simulink model "ConSys_A1"  (Simulink 8.3)
settings: Solver=ode3  StartTime=0.0  StopTime=Time(end)  FixedStep=Ts  RelTol=1e-3
values from neighbouring files (symbols this model uses):
  d = r*h    (= 1.6)    [StartUp_A1.m]
  d0 = d*h    (= 0.0032)    [StartUp_A1.m]
  h = 0.002    [StartUp_A1.m]
  Ka = diag([ 3  20  20  150  355  520])    [StartUp_A1.m]
  Kd = diag([ 3   5  25  100   15 1050])    [StartUp_A1.m]
  Ki = diag([35 555 810 7410 1850 5815])    [StartUp_A1.m]
  Kp = diag([55 180 350 1960  680 4450])    [StartUp_A1.m]
  r = 800    [StartUp_A1.m]
  TD = ss(Atd,Btd,Ctd,Dtd,Ts)    [StartUp_A1.m]
  Ts = 1/200    (= 0.005)    [StartUp_A1.m]
undefined symbols (not defined in the file or in its folder): DiscIntNeverNeededParam
undefined symbols (not defined in the file): ADAMS_cwd, ADAMS_exec, ADAMS_host, ADAMS_init, ADAMS_inputs, ADAMS_outputs, ADAMS_prefix, ADAMS_static, ADAMS_sysdir
libraries: cstblocks x6
(part 6 of 9)

== matlab function A2/MATLAB Function 3 ==
  data: q input double; V3 output double; dq input double
function V3 = V3(q,dq)
%#codegen
Th1=q(1,1); Th2=q(2,1); Th3=q(3,1); Th4=q(4,1); Th5=q(5,1); Th6=q(6,1);
dTh1=dq(1); dTh2=dq(2); dTh3=dq(3); dTh4=dq(4); dTh5=dq(5); dTh6=dq(6);
%---------------------------
V311=(1.3719*sin(2.0*Th2 + 2.0*Th3) - 0.006265*cos(2.0*Th2 + 2.0*Th3) + (0.01602*cos(Th2 + Th3) + 2.4568*sin(Th2 + Th3))*(0.13649*cos(Th2 + Th3) - 0.00089*sin(Th2 + Th3) + 0.36*sin(Th2) - 0.07) - 0.5*(cos(Th6)*(sin(Th2 + Th3)*sin(Th5) - 1.0*cos(Th2 + Th3)*cos(Th4)*cos(Th5)) + cos(Th2 + Th3)*sin(Th4)*sin(Th6))*(0.001043*cos(Th6)*(cos(Th2 + Th3)*sin(Th5) + sin(Th2 + Th3)*cos(Th4)*cos(Th5)) - 4.0e-6*cos(Th2 + Th3)*cos(Th5) + 4.0e-6*sin(Th2 + Th3)*cos(Th4)*sin(Th5) - 0.001043*sin(Th2 + Th3)*sin(Th4)*sin(Th6)) - 1.0*(0.126*sin(Th2 + Th3) + 0.00062*cos(Th2 + Th3)*sin(Th4) - 0.00152*sin(Th2 + Th3)*cos(Th5) - 0.00002*sin(Th2 + Th3)*sin(Th5) + 0.254*cos(Th2)*sin(Th3) + 0.254*cos(Th3)*sin(Th2) + 0.00002*cos(Th2 + Th3)*cos(Th4)*cos(Th5) - 0.00152*cos(Th2 + Th3)*cos(Th4)*sin(Th5))*(0.36*sin(Th2) - 0.126*cos(Th2 + Th3) + 0.00152*cos(Th2 + Th3)*cos(Th5) + 0.00002*cos(Th2 + Th3)*sin(Th5) + 0.00062*sin(Th2 + Th3)*sin(Th4) - 0.254*cos(Th2)*cos(Th3) + 0.254*sin(Th2)*sin(Th3) + 0.00002*sin(Th2 + Th3)*cos(Th4)*cos(Th5) - 0.00152*sin(Th2 + Th3)*cos(Th4)*sin(Th5) - 0.07) + (0.063*sin(Th2 + Th3) + 0.02603*sin(Th2 + Th3)*cos(Th5) + 0.127*cos(Th2)*sin(Th3) + 0.127*cos(Th3)*sin(Th2) + 0.02603*cos(Th2 + Th3)*cos(Th4)*sin(Th5) + 0.000115*cos(Th2 + Th3)*sin(Th4)*sin(Th6) + 0.000115*sin(Th2 + Th3)*cos(Th6)*sin(Th5) - 0.000115*cos(Th2 + Th3)*cos(Th4)*cos(Th5)*cos(Th6))*(0.126*cos(Th2 + Th3) - 0.36*sin(Th2) + 0.05206*cos(Th2 + Th3)*cos(Th5) + 0.254*cos(Th2)*cos(Th3) - 0.254*sin(Th2)*sin(Th3) + 0.00023*cos(Th2 + Th3)*cos(Th6)*sin(Th5) - 0.05206*sin(Th2 + Th3)*cos(Th4)*sin(Th5) - 0.00023*sin(Th2 + Th3)*sin(Th4)*sin(Th6) + 0.00023*sin(Th2 + Th3)*cos(Th4)*cos(Th5)*cos(Th6) + 0.07) - 0.004943*cos(Th2 + Th3)*sin(Th2 + Th3) - 0.5*(sin(Th6)*(cos(Th2 + Th3)*sin(Th5) + sin(Th2 + Th3)*cos(Th4)*cos(Th5)) + sin(Th2 + Th3)*cos(Th6)*sin(Th4))*(0.00104*sin(Th6)*(sin(Th2 + Th3)*sin(Th5) - 1.0*cos(Th2 + Th3)*cos(Th4)*cos(Th5)) - 0.00104*cos(Th2 + Th3)*cos(Th6)*sin(Th4)) - 0.5*(sin(Th6)*(sin(Th2 + Th3)*sin(Th5) - 1.0*cos(Th2 + Th3)*cos(Th4)*cos(Th5)) - 1.0*cos(Th2 + Th3)*cos(Th6)*sin(Th4))*(0.00104*sin(Th6)*(cos(Th2 + Th3)*sin(Th5) + sin(Th2 + Th3)*cos(Th4)*cos(Th5)) + 0.00104*sin(Th2 + Th3)*cos(Th6)*sin(Th4)) + 0.5*(sin(Th2 + Th3)*cos(Th5) + cos(Th2 + Th3)*cos(Th4)*sin(Th5))*(4.0e-6*cos(Th6)*(cos(Th2 + Th3)*sin(Th5) + sin(Th2 + Th3)*cos(Th4)*cos(Th5)) - 0.000116*cos(Th2 + Th3)*cos(Th5) + 0.000116*sin(Th2 + Th3)*cos(Th4)*sin(Th5) - 4.0e-6*sin(Th2 + Th3)*sin(Th4)*sin(Th6)) + 0.5*(cos(Th2 + Th3)*cos(Th5) - 1.0*sin(Th2 + Th3)*cos(Th4)*sin(Th5))*(4.0e-6*cos(Th6)*(sin(Th2 + Th3)*sin(Th5) - 1.0*cos(Th2 + Th3)*cos(Th4)*cos(Th5)) - 0.000116*sin(Th2 + Th3)*cos(Th5) - 0.000116*cos(Th2 + Th3)*cos(Th4)*sin(Th5) + 4.0e-6*cos(Th2 + Th3)*sin(Th4)*sin(Th6)) + (0.55399*sin(Th2 + Th3) + 1.651*cos(Th2)*sin(Th3) + 1.651*cos(Th3)*sin(Th2))*(0.08523*cos(Th2 + Th3) - 0.36*sin(Th2) + 0.254*cos(Th2)*cos(Th3) - 0.254*sin(Th2)*sin(Th3) + 0.07) - 0.5*(cos(Th6)*(cos(Th2 + Th3)*sin(Th5) + sin(Th2 + Th3)*cos(Th4)*cos(Th5)) - 1.0*sin(Th2 + Th3)*sin(Th4)*sin(Th6))*(0.001043*cos(Th6)*(sin(Th2 + Th3)*sin(Th5) - 1.0*cos(Th2 + Th3)*cos(Th4)*cos(Th5)) - 4.0e-6*sin(Th2 + Th3)*cos(Th5) - 4.0e-6*cos(Th2 + Th3)*cos(Th4)*sin(Th5) + 0.001043*cos(Th2 + Th3)*sin(Th4)*sin(Th6)) + 0.011125*cos(Th2 + Th3)*sin(Th2 + Th3)*cos(Th4)^2 - 0.000489*cos(Th2 + Th3)*sin(Th2 + Th3)*cos(Th5)^2 + 0.02091*cos(Th2 + Th3)*sin(Th2 + Th3)*sin(Th4)^2 - 0.004898*cos(Th2 + Th3)*sin(Th2 + Th3)*sin(Th5)^2 + 0.00004*cos(Th2 + Th3)^2*cos(Th5)*sin(Th4) - 0.00004*sin(Th2 + Th3)^2*cos(Th5)*sin(Th4) + 0.004409*cos(Th2 + Th3)^2*cos(Th4)*cos(Th5)*sin(Th5) - 0.004409*sin(Th2 + Th3)^2*cos(Th4)*cos(Th5)*sin(Th5) + 0.004898*cos(Th2 + Th3)*sin(Th2 + Th3)*cos(Th4)^2*cos(Th5)^2 + 0.000489*cos(Th2 + Th3)*sin(Th2 + Th3)*cos(Th4)^2*sin(Th5)^2 - 0.00008*cos(Th2 + Th3)*sin(Th2 + Th3)*cos(Th4)*sin(Th4)*sin(Th5))*dTh1*dTh1;
O312=0.019809*cos(Th2 + Th3) - 0.000076053*sin(Th2 + Th3) - 0.5*(0.00062*cos(Th4) - 0.00002*cos(Th5)*sin(Th4) + 0.00152*sin(Th4)*sin(Th5))*(0.00152*cos(Th2 + Th3)*cos(Th5) - 0.126*cos(Th2 + Th3) + 0.00002*cos(Th2 + Th3)*sin(Th5) + 0.00062*sin(Th2 + Th3)*sin(Th4) - 0.254*cos(Th2)*cos(Th3) + 0.254*sin(Th2)*sin(Th3) + 0.00002*sin(Th2 + Th3)*cos(Th4)*cos(Th5) - 0.00152*sin(Th2 + Th3)*cos(Th4)*sin(Th5)) + 0.00002*sin(Th2 + Th3)*sin(Th5) + 0.5*(0.000115*cos(Th4)*sin(Th6) - 0.02603*sin(Th4)*sin(Th5) + 0.000115*cos(Th5)*cos(Th6)*sin(Th4))*(0.126*cos(Th2 + Th3) + 0.05206*cos(Th2 + Th3)*cos(Th5) + 0.254*cos(Th2)*cos(Th3) - 0.254*sin(Th2)*sin(Th3) + 0.00023*cos(Th2 + Th3)*cos(Th6)*sin(Th5) - 0.05206*sin(Th2 + Th3)*cos(Th4)*sin(Th5) - 0.00023*sin(Th2 + Th3)*sin(Th4)*sin(Th6) + 0.00023*sin(Th2 + Th3)*cos(Th4)*cos(Th5)*cos(Th6)) + 0.00002*cos(Th2 + Th3)*cos(Th4)*cos(Th5) - 2.0e-6*cos(Th2 + Th3)*cos(Th6)*sin(Th4) + 0.0051115*sin(Th2 + Th3)*cos(Th4)*sin(Th4) + 2.0e-6*sin(Th2 + Th3)*sin(Th5)*sin(Th6) - 0.00004*sin(Th2 + Th3)*cos(Th4)^2*sin(Th5) + 2.0e-6*cos(Th2 + Th3)*cos(Th4)*cos(Th5)*sin(Th6) - 0.0026665*cos(Th2 + Th3)*cos(Th5)*sin(Th4)*sin(Th5) + 1.5e-6*sin(Th2 + Th3)*cos(Th5)*cos(Th6)*sin(Th6) + 4.0e-6*cos(Th2 + Th3)*cos(Th5)^2*cos(Th6)*sin(Th4) - 0.0026665*sin(Th2 + Th3)*cos(Th4)*cos(Th5)^2*sin(Th4) - 1.5e-6*sin(Th2 + Th3)*cos(Th4)*cos(Th6)^2*sin(Th4) - 4.0e-6*sin(Th2 + Th3)*cos(Th4)^2*sin(Th5)*sin(Th6) - 1.5e-6*cos(Th2 + Th3)*cos(Th5)*cos(Th6)^2*sin(Th4)*sin(Th5) - 3.0e-6*sin(Th2 + Th3)*cos(Th4)^2*cos(Th5)*cos(Th6)*sin(Th6) - 1.5e-6*sin(Th2 + Th3)*cos(Th4)*cos(Th5)^2*cos(Th6)^2*sin(Th4) - 1.5e-6*cos(Th2 + Th3)*cos(Th4)*cos(Th6)*sin(Th5)*sin(Th6) - 4.0e-6*sin(Th2 + Th3)*cos(Th4)*cos(Th5)*cos(Th6)*sin(Th4)*sin(Th5);
V312=O312*dTh1*dTh2;
V313=O312*dTh1*dTh3;
V314=(0.0054606*cos(Th2)*cos(Th3) - 0.0054606*sin(Th2)*sin(Th3) + 0.02316*cos(Th4)^2*sin(Th2)*sin(Th3) + 0.0033452*cos(Th5)^2*sin(Th2)*sin(Th3) + 4.4603e-6*cos(Th6)^2*sin(Th2)*sin(Th3) - 4.56e-8*cos(Th2)*cos(Th4)*sin(Th3) - 4.56e-8*cos(Th3)*cos(Th4)*sin(Th2) - 0.0003534*cos(Th2)*sin(Th3)*sin(Th4) - 0.0003534*cos(Th3)*sin(Th2)*sin(Th4) - 0.02316*cos(Th2)*cos(Th3)*cos(Th4)^2 - 0.0033452*cos(Th2)*cos(Th3)*cos(Th5)^2 - 4.4603e-6*cos(Th2)*cos(Th3)*cos(Th6)^2 - 0.013381*cos(Th4)^2*cos(Th5)^2*sin(Th2)*sin(Th3) - 5.9471e-6*cos(Th4)^2*cos(Th6)^2*sin(Th2)*sin(Th3) + 1.4868e-6*cos(Th5)^2*cos(Th6)^2*sin(Th2)*sin(Th3) - 0.0000114*cos(Th2)*cos(Th4)*cos(Th5)*sin(Th3) - 0.0000114*cos(Th3)*cos(Th4)*cos(Th5)*sin(Th2) - 3.04e-8*cos(Th2)*cos(Th3)*cos(Th5)*sin(Th5) - 0.00001498*cos(Th2)*cos(Th4)*cos(Th6)*sin(Th3) - 0.00001498*cos(Th3)*cos(Th4)*cos(Th6)*sin(Th2) - 0.013971*cos(Th2)*cos(Th4)*sin(Th3)*sin(Th5) - 0.000058586*cos(Th2)*cos(Th5)*sin(Th3)*sin(Th4) - 0.013971*cos(Th3)*cos(Th4)*sin(Th2)*sin(Th5) - 0.000058586*cos(Th3)*cos(Th5)*sin(Th2)*sin(Th4) + 1.86e-8*cos(Th2)*sin(Th3)*sin(Th4)*sin(Th5) + 1.86e-8*cos(Th3)*sin(Th2)*sin(Th4)*sin(Th5) - 0.00006555*cos(Th2)*sin(Th3)*sin(Th4)*sin(Th6) - 0.00006555*cos(Th3)*sin(Th2)*sin(Th4)*sin(Th6) + 3.04e-8*cos(Th5)*sin(Th2)*sin(Th3)*sin(Th5) + 9.12e-8*cos(Th2)*cos(Th4)*cos(Th5)^2*sin(Th3) + 9.12e-8*cos(Th3)*cos(Th4)*cos(Th5)^2*sin(Th2) + 0.013381*cos(Th2)*cos(Th3)*cos(Th4)^2*cos(Th5)^2 + 5.9471e-6*cos(Th2)*cos(Th3)*cos(Th4)^2*cos(Th6)^2 - 1.4868e-6*cos(Th2)*cos(Th3)*cos(Th5)^2*cos(Th6)^2 - 4.96e-8*cos(Th2)*cos(Th3)*cos(Th4)*cos(Th5)*sin(Th4) + 0.00006555*cos(Th2)*cos(Th4)*cos(Th5)*cos(Th6)*sin(Th3) + 0.00006555*cos(Th3)*cos(Th4)*cos(Th5)*cos(Th6)*sin(Th2) - 9.9869e-6*cos(Th2)*cos(Th3)*cos(Th5)*cos(Th6)*sin(Th5) + 5.9471e-6*cos(Th2)*cos(Th3)*cos(Th4)^2*cos(Th5)^2*cos(Th6)^2 - 0.00015623*cos(Th2)*cos(Th3)*cos(Th4)*sin(Th4)*sin(Th5) - 0.010036*cos(Th2)*cos(Th4)*cos(Th5)*sin(Th3)*sin(Th5) - 0.010036*cos(Th3)*cos(Th4)*cos(Th5)*sin(Th2)*sin(Th5) + 4.96e-8*cos(Th4)*cos(Th5)*sin(Th2)*sin(Th3)*sin(Th4) - 0.00001498*cos(Th2)*cos(Th5)*sin(Th3)*sin(Th4)*sin(Th6) - 0.00001498*cos(Th3)*cos(Th5)*sin(Th2)*sin(Th4)*sin(Th6) + 9.9869e-6*cos(Th5)*cos(Th6)*sin(Th2)*sin(Th3)*sin(Th5) - 5.9471e-6*cos(Th4)^2*cos(Th5)^2*cos(Th6)^2*sin(Th2)*sin(Th3) + 0.00015623*cos(Th4)*sin(Th2)*sin(Th3)*sin(Th4)*sin(Th5) + 1.216e-7*cos(Th2)*cos(Th3)*cos(Th4)^2*cos(Th5)*sin(Th5) + 0.000029961*cos(Th2)*cos(Th4)*cos(Th5)^2*cos(Th6)*sin(Th3) + 0.000029961*cos(Th3)*cos(Th4)*cos(Th5)^2*cos(Th6)*sin(Th2) - 1.216e-7*cos(Th4)^2*cos(Th5)*sin(Th2)*sin(Th3)*sin(Th5) + 0.000039948*cos(Th2)*cos(Th3)*cos(Th4)^2*cos(Th5)*cos(Th6)*sin(Th5) - 4.4603e-6*cos(Th2)*cos(Th4)*cos(Th5)*cos(Th6)^2*sin(Th3)*sin(Th5) - 4.4603e-6*cos(Th3)*cos(Th4)*cos(Th5)*cos(Th6)^2*sin(Th2)*sin(Th5) - 0.000039948*cos(Th4)^2*cos(Th5)*cos(Th6)*sin(Th2)*sin(Th3)*sin(Th5) - 0.000039948*cos(Th2)*cos(Th3)*cos(Th4)*sin(Th4)*sin(Th5)*sin(Th6) + 4.4603e-6*cos(Th2)*cos(Th6)*sin(Th3)*sin(Th4)*sin(Th5)*sin(Th6) + 4.4603e-6*cos(Th3)*cos(Th6)*sin(Th2)*sin(Th4)*sin(Th5)*sin(Th6) + 0.000039948*cos(Th4)*sin(Th2)*sin(Th3)*sin(Th4)*sin(Th5)*sin(Th6) - 0.000011894*cos(Th2)*cos(Th3)*cos(Th4)*cos(Th5)*cos(Th6)*sin(Th4)*sin(Th6) + 0.000011894*cos(Th4)*cos(Th5)*cos(Th6)*sin(Th2)*sin(Th3)*sin(Th4)*sin(Th6))*dTh1*dTh4;
V315=(1.86e-8*cos(Th2)*cos(Th3)*sin(Th5) - 0.000058586*cos(Th2)*cos(Th3)*cos(Th5) + 0.0028942*cos(Th2)*sin(Th3)*sin(Th4) + 0.0028942*cos(Th3)*sin(Th2)*sin(Th4) + 0.000058586*cos(Th5)*sin(Th2)*sin(Th3) - 1.86e-8*sin(Th2)*sin(Th3)*sin(Th5) - 6.08e-8*cos(Th2)*cos(Th3)*cos(Th4)*sin(Th4) - 6.2e-9*cos(Th2)*cos(Th4)*cos(Th5)*sin(Th3) - 6.2e-9*cos(Th3)*cos(Th4)*cos(Th5)*sin(Th2) - 0.00001498*cos(Th2)*cos(Th3)*cos(Th5)*sin(Th6) - 0.000019529*cos(Th2)*cos(Th4)*sin(Th3)*sin(Th5) - 0.013971*cos(Th2)*cos(Th5)*sin(Th3)*sin(Th4) - 0.000019529*cos(Th3)*cos(Th4)*sin(Th2)*sin(Th5) - 0.013971*cos(Th3)*cos(Th5)*sin(Th2)*sin(Th4) + 6.08e-8*cos(Th4)*sin(Th2)*sin(Th3)*sin(Th4) + 0.0000114*cos(Th2)*sin(Th3)*sin(Th4)*sin(Th5) + 0.0000114*cos(Th3)*sin(Th2)*sin(Th4)*sin(Th5) + 0.00001498*cos(Th5)*sin(Th2)*sin(Th3)*sin(Th6) + 0.000078115*cos(Th2)*cos(Th3)*cos(Th4)^2*cos(Th5) - 2.48e-8*cos(Th2)*cos(Th3)*cos(Th4)^2*sin(Th5) - 0.013381*cos(Th2)*cos(Th5)^2*sin(Th3)*sin(Th4) - 0.013381*cos(Th3)*cos(Th5)^2*sin(Th2)*sin(Th4) - 0.000078115*cos(Th4)^2*cos(Th5)*sin(Th2)*sin(Th3) + 4.4603e-6*cos(Th2)*cos(Th6)^2*sin(Th3)*sin(Th4) + 4.4603e-6*cos(Th3)*cos(Th6)^2*sin(Th2)*sin(Th4) + 2.48e-8*cos(Th4)^2*sin(Th2)*sin(Th3)*sin(Th5) - 0.000019974*cos(Th2)*cos(Th3)*cos(Th4)*cos(Th6)*sin(Th4) + 4.4603e-6*cos(Th2)*cos(Th3)*cos(Th6)*sin(Th5)*sin(Th6) - 1.216e-7*cos(Th2)*cos(Th5)*sin(Th3)*sin(Th4)*sin(Th5) - 1.216e-7*cos(Th3)*cos(Th5)*sin(Th2)*sin(Th4)*sin(Th5) + 0.000019974*cos(Th4)*cos(Th6)*sin(Th2)*sin(Th3)*sin(Th4) - 4.9934e-6*cos(Th2)*cos(Th4)*sin(Th3)*sin(Th5)*sin(Th6) - 0.00006555*cos(Th2)*cos(Th6)*sin(Th3)*sin(Th4)*sin(Th5) - 4.9934e-6*cos(Th3)*cos(Th4)*sin(Th2)*sin(Th5)*sin(Th6) - 0.00006555*cos(Th3)*cos(Th6)*sin(Th2)*sin(Th4)*sin(Th5) - 4.4603e-6*cos(Th6)*sin(Th2)*sin(Th3)*sin(Th5)*sin(Th6) + 1.216e-7*cos(Th2)*cos(Th3)*cos(Th4)*cos(Th5)^2*sin(Th4) + 0.000019974*cos(Th2)*cos(Th3)*cos(Th4)^2*cos(Th5)*sin(Th6) - 1.216e-7*cos(Th4)*cos(Th5)^2*sin(Th2)*sin(Th3)*sin(Th4) - 0.000019974*cos(Th4)^2*cos(Th5)*sin(Th2)*sin(Th3)*sin(Th6) - 5.9471e-6*cos(Th2)*cos(Th5)^2*cos(Th6)^2*sin(Th3)*sin(Th4) - 5.9471e-6*cos(Th3)*cos(Th5)^2*cos(Th6)^2*sin(Th2)*sin(Th4) + 0.000039948*cos(Th2)*cos(Th3)*cos(Th4)*cos(Th5)^2*cos(Th6)*sin(Th4) - 5.9471e-6*cos(Th2)*cos(Th3)*cos(Th4)^2*cos(Th6)*sin(Th5)*sin(Th6) - 0.000039948*cos(Th4)*cos(Th5)^2*cos(Th6)*sin(Th2)*sin(Th3)*sin(Th4) + 5.9471e-6*cos(Th4)^2*cos(Th6)*sin(Th2)*sin(Th3)*sin(Th5)*sin(Th6) - 0.013381*cos(Th2)*cos(Th3)*cos(Th4)*cos(Th5)*sin(Th4)*sin(Th5) - 1.4868e-6*cos(Th2)*cos(Th4)*cos(Th5)*cos(Th6)*sin(Th3)*sin(Th6) - 1.4868e-6*cos(Th3)*cos(Th4)*cos(Th5)*cos(Th6)*sin(Th2)*sin(Th6) - 0.000039948*cos(Th2)*cos(Th5)*cos(Th6)*sin(Th3)*sin(Th4)*sin(Th5) - 0.000039948*cos(Th3)*cos(Th5)*cos(Th6)*sin(Th2)*sin(Th4)*sin(Th5) + 0.013381*cos(Th4)*cos(Th5)*sin(Th2)*sin(Th3)*sin(Th4)*sin(Th5) + 5.9471e-6*cos(Th4)*cos(Th5)*cos(Th6)^2*sin(Th2)*sin(Th3)*sin(Th4)*sin(Th5) - 5.9471e-6*cos(Th2)*cos(Th3)*cos(Th4)*cos(Th5)*cos(Th6)^2*sin(Th4)*sin(Th5))*dTh1*dTh5;
V316=(0.00005504*cos(Th5)*sin(Th2)*sin(Th3) - 0.00005504*cos(Th2)*cos(Th3)*cos(Th5) + 0.00006555*cos(Th2)*cos(Th4)*cos(Th6)*sin(Th3) + 0.00006555*cos(Th3)*cos(Th4)*cos(Th6)*sin(Th2) - 4.9934e-6*cos(Th2)*cos(Th3)*cos(Th6)*sin(Th5) + 0.000060987*cos(Th2)*cos(Th4)*sin(Th3)*sin(Th5) + 0.000060987*cos(Th3)*cos(Th4)*sin(Th2)*sin(Th5) + 4.9934e-6*cos(Th2)*sin(Th3)*sin(Th4)*sin(Th6) + 4.9934e-6*cos(Th3)*sin(Th2)*sin(Th4)*sin(Th6) + 4.9934e-6*cos(Th6)*sin(Th2)*sin(Th3)*sin(Th5) - 5.9471e-6*cos(Th2)*cos(Th3)*cos(Th4)^2*cos(Th5) - 5.9471e-6*cos(Th2)*cos(Th3)*cos(Th5)*cos(Th6)^2 + 5.9471e-6*cos(Th4)^2*cos(Th5)*sin(Th2)*sin(Th3) + 5.9471e-6*cos(Th5)*cos(Th6)^2*sin(Th2)*sin(Th3) + 0.00001498*cos(Th2)*cos(Th4)*cos(Th5)*cos(Th6)*sin(Th3) + 0.00001498*cos(Th3)*cos(Th4)*cos(Th5)*cos(Th6)*sin(Th2) - 0.00006555*cos(Th2)*cos(Th5)*sin(Th3)*sin(Th4)*sin(Th6) - 0.00006555*cos(Th3)*cos(Th5)*sin(Th2)*sin(Th4)*sin(Th6) + 0.000019974*cos(Th2)*cos(Th3)*cos(Th4)^2*cos(Th6)*sin(Th5) - 5.9471e-6*cos(Th2)*cos(Th4)*cos(Th6)^2*sin(Th3)*sin(Th5) - 5.9471e-6*cos(Th3)*cos(Th4)*cos(Th6)^2*sin(Th2)*sin(Th5) - 0.000019974*cos(Th2)*cos(Th5)^2*sin(Th3)*sin(Th4)*sin(Th6) - 0.000019974*cos(Th3)*cos(Th5)^2*sin(Th2)*sin(Th4)*sin(Th6) - 0.000019974*cos(Th4)^2*cos(Th6)*sin(Th2)*sin(Th3)*sin(Th5) + 0.000011894*cos(Th2)*cos(Th3)*cos(Th4)^2*cos(Th5)*cos(Th6)^2 - 0.000011894*cos(Th4)^2*cos(Th5)*cos(Th6)^2*sin(Th2)*sin(Th3) - 5.9471e-6*cos(Th2)*cos(Th3)*cos(Th4)*cos(Th6)*sin(Th4)*sin(Th6) + 5.9471e-6*cos(Th4)*cos(Th6)*sin(Th2)*sin(Th3)*sin(Th4)*sin(Th6) + 5.9471e-6*cos(Th4)*cos(Th5)^2*cos(Th6)*sin(Th2)*sin(Th3)*sin(Th4)*sin(Th6) - 0.000019974*cos(Th2)*cos(Th3)*cos(Th4)*cos(Th5)*sin(Th4)*sin(Th5)*sin(Th6) + 5.9471e-6*cos(Th2)*cos(Th5)*cos(Th6)*sin(Th3)*sin(Th4)*sin(Th5)*sin(Th6) + 5.9471e-6*cos(Th3)*cos(Th5)*cos(Th6)*sin(Th2)*sin(Th4)*sin(Th5)*sin(Th6) + 0.000019974*cos(Th4)*cos(Th5)*sin(Th2)*sin(Th3)*sin(Th4)*sin(Th5)*sin(Th6) - 5.9471e-6*cos(Th2)*cos(Th3)*cos(Th4)*cos(Th5)^2*cos(Th6)*sin(Th4)*sin(Th6))*dTh1*dTh6;
%---------------------------
V321=(0.000076053*sin(Th2 + Th3) - 0.019809*cos(Th2 + Th3) + 0.5*(0.00062*cos(Th4) - 0.00002*cos(Th5)*sin(Th4) + 0.00152*sin(Th4)*sin(Th5))*(0.00152*cos(Th2 + Th3)*cos(Th5) - 0.126*cos(Th2 + Th3) + 0.00002*cos(Th2 + Th3)*sin(Th5) + 0.00062*sin(Th2 + Th3)*sin(Th4) - 0.254*cos(Th2)*cos(Th3) + 0.254*sin(Th2)*sin(Th3) + 0.00002*sin(Th2 + Th3)*cos(Th4)*cos(Th5) - 0.00152*sin(Th2 + Th3)*cos(Th4)*sin(Th5)) - 0.00002*sin(Th2 + Th3)*sin(Th5) - 0.5*(0.000115*cos(Th4)*sin(Th6) - 0.02603*sin(Th4)*sin(Th5) + 0.000115*cos(Th5)*cos(Th6)*sin(Th4))*(0.126*cos(Th2 + Th3) + 0.05206*cos(Th2 + Th3)*cos(Th5) + 0.254*cos(Th2)*cos(Th3) - 0.254*sin(Th2)*sin(Th3) + 0.00023*cos(Th2 + Th3)*cos(Th6)*sin(Th5) - 0.05206*sin(Th2 + Th3)*cos(Th4)*sin(Th5) - 0.00023*sin(Th2 + Th3)*sin(Th4)*sin(Th6) + 0.00023*sin(Th2 + Th3)*cos(Th4)*cos(Th5)*cos(Th6)) - 0.00002*cos(Th2 + Th3)*cos(Th4)*cos(Th5) + 2.0e-6*cos(Th2 + Th3)*cos(Th6)*sin(Th4) - 0.0051115*sin(Th2 + Th3)*cos(Th4)*sin(Th4) - 2.0e-6*sin(Th2 + Th3)*sin(Th5)*sin(Th6) + 0.00004*sin(Th2 + Th3)*cos(Th4)^2*sin(Th5) - 2.0e-6*cos(Th2 + Th3)*cos(Th4)*cos(Th5)*sin(Th6) + 0.0026665*cos(Th2 + Th3)*cos(Th5)*sin(Th4)*sin(Th5) - 1.5e-6*sin(Th2 + Th3)*cos(Th5)*cos(Th6)*sin(Th6) - 4.0e-6*cos(Th2 + Th3)*cos(Th5)^2*cos(Th6)*sin(Th4) + 0.0026665*sin(Th2 + Th3)*cos(Th4)*cos(Th5)^2*sin(Th4) + 1.5e-6*sin(Th2 + Th3)*cos(Th4)*cos(Th6)^2*sin(Th4) + 4.0e-6*sin(Th2 + Th3)*cos(Th4)^2*sin(Th5)*sin(Th6) + 1.5e-6*cos(Th2 + Th3)*cos(Th5)*cos(Th6)^2*sin(Th4)*sin(Th5) + 3.0e-6*sin(Th2 + Th3)*cos(Th4)^2*cos(Th5)*cos(Th6)*sin(Th6) + 1.5e-6*sin(Th2 + Th3)*cos(Th4)*cos(Th5)^2*cos(Th6)^2*sin(Th4) + 1.5e-6*cos(Th2 + Th3)*cos(Th4)*cos(Th6)*sin(Th5)*sin(Th6) + 4.0e-6*sin(Th2 + Th3)*cos(Th4)*cos(Th5)*cos(Th6)*sin(Th4)*sin(Th5))*dTh2*dTh1;
V322=(7.2e-6*cos(Th3)*sin(Th5) - 0.0057672*sin(Th3) - 0.0088236*cos(Th3)*cos(Th5) - 0.11454*cos(Th3) + 0.0002232*sin(Th3)*sin(Th4) + 7.2e-6*cos(Th4)*cos(Th5)*sin(Th3) - 0.0000414*cos(Th3)*cos(Th6)*sin(Th5) + 0.0088236*cos(Th4)*sin(Th3)*sin(Th5) + 0.0000414*sin(Th3)*sin(Th4)*sin(Th6) - 0.0000414*cos(Th4)*cos(Th5)*cos(Th6)*sin(Th3))*dTh2*dTh2;
V323=(0.057271*cos(Th3) + 0.0028836*sin(Th3) + 0.0044118*cos(Th3)*cos(Th5) - 3.6e-6*cos(Th3)*sin(Th5) - 0.0001116*sin(Th3)*sin(Th4) - 3.6e-6*cos(Th4)*cos(Th5)*sin(Th3) + 0.0000207*cos(Th3)*cos(Th6)*sin(Th5) - 0.0044118*cos(Th4)*sin(Th3)*sin(Th5) - 0.0000207*sin(Th3)*sin(Th4)*sin(Th6) + 0.0000207*cos(Th4)*cos(Th5)*cos(Th6)*sin(Th3))*dTh2*dTh3;
V324=(4.96e-8*cos(Th4)^2*cos(Th5) - 2.48e-8*cos(Th5) - 0.000078115*sin(Th5) - 0.01158*sin(2.0*Th4) + 0.00015623*cos(Th4)^2*sin(Th5) + 0.0001116*cos(Th3)*cos(Th4) - 0.000019974*sin(Th5)*sin(Th6) + 0.000039948*cos(Th4)^2*sin(Th5)*sin(Th6) - 3.6e-6*cos(Th3)*cos(Th5)*sin(Th4) + 0.0000207*cos(Th3)*cos(Th4)*sin(Th6) - 5.9471e-6*cos(Th5)*cos(Th6)*sin(Th6) - 0.0044118*cos(Th3)*sin(Th4)*sin(Th5) + 0.013381*cos(Th4)*cos(Th5)^2*sin(Th4) + 5.9471e-6*cos(Th4)*cos(Th6)^2*sin(Th4) + 5.9471e-6*cos(Th4)*cos(Th5)^2*cos(Th6)^2*sin(Th4) + 0.0000207*cos(Th3)*cos(Th5)*cos(Th6)*sin(Th4) + 1.216e-7*cos(Th4)*cos(Th5)*sin(Th4)*sin(Th5) + 0.000011894*cos(Th4)^2*cos(Th5)*cos(Th6)*sin(Th6) + 0.000039948*cos(Th4)*cos(Th5)*cos(Th6)*sin(Th4)*sin(Th5))*dTh2*dTh4;
V325=(6.08e-8*cos(Th4)^2 - 0.0000152*cos(Th5) - 0.000019974*cos(Th6) - 0.018628*sin(Th5) - 0.0066904*sin(2.0*Th5) + 1.216e-7*cos(Th5)^2 + 0.000019974*cos(Th4)^2*cos(Th6) + 0.000039948*cos(Th5)^2*cos(Th6) - 1.216e-7*cos(Th4)^2*cos(Th5)^2 + 0.0000874*cos(Th5)*cos(Th6) - 3.6e-6*cos(Th5)*sin(Th3) - 0.0044118*sin(Th3)*sin(Th5) - 0.000039948*cos(Th4)^2*cos(Th5)^2*cos(Th6) + 0.0044118*cos(Th3)*cos(Th4)*cos(Th5) - 3.6e-6*cos(Th3)*cos(Th4)*sin(Th5) + 0.000078115*cos(Th4)*cos(Th5)*sin(Th4) + 0.0000207*cos(Th5)*cos(Th6)*sin(Th3) - 2.48e-8*cos(Th4)*sin(Th4)*sin(Th5) + 0.013381*cos(Th4)^2*cos(Th5)*sin(Th5) - 5.9471e-6*cos(Th5)*cos(Th6)^2*sin(Th5) + 5.9471e-6*cos(Th4)^2*cos(Th5)*cos(Th6)^2*sin(Th5) + 0.0000207*cos(Th3)*cos(Th4)*cos(Th6)*sin(Th5) + 0.000019974*cos(Th4)*cos(Th5)*sin(Th4)*sin(Th6) - 5.9471e-6*cos(Th4)*cos(Th6)*sin(Th4)*sin(Th5)*sin(Th6) - 6.08e-8)*dTh2*dTh5;
V326=(0.0000207*cos(Th3)*cos(Th6)*sin(Th4) - 0.0000874*sin(Th5)*sin(Th6) - 5.9471e-6*cos(Th4)*cos(Th5)*sin(Th4) - 0.000019974*cos(Th5)*sin(Th5)*sin(Th6) - 0.0000207*sin(Th3)*sin(Th5)*sin(Th6) + 5.9471e-6*cos(Th4)^2*cos(Th6)*sin(Th6) - 5.9471e-6*cos(Th5)^2*cos(Th6)*sin(Th6) + 5.9471e-6*cos(Th4)^2*cos(Th5)^2*cos(Th6)*sin(Th6) + 0.0000207*cos(Th3)*cos(Th4)*cos(Th5)*sin(Th6) + 0.000019974*cos(Th4)*cos(Th6)*sin(Th4)*sin(Th5) + 0.000011894*cos(Th4)*cos(Th5)*cos(Th6)^2*sin(Th4) + 0.000019974*cos(Th4)^2*cos(Th5)*sin(Th5)*sin(Th6))*dTh2*dTh6;
%---------------------------
V331=(0.000076053*sin(Th2 + Th3) - 0.019809*cos(Th2 + Th3) + 0.5*(0.00062*cos(Th4) - 0.00002*cos(Th5)*sin(Th4) + 0.00152*sin(Th4)*sin(Th5))*(0.00152*cos(Th2 + Th3)*cos(Th5) - 0.126*cos(Th2 + Th3) + 0.00002*cos(Th2 + Th3)*sin(Th5) + 0.00062*sin(Th2 + Th3)*sin(Th4) - 0.254*cos(Th2)*cos(Th3) + 0.254*sin(Th2)*sin(Th3) + 0.00002*sin(Th2 + Th3)*cos(Th4)*cos(Th5) - 0.00152*sin(Th2 + Th3)*cos(Th4)*sin(Th5)) - 0.00002*sin(Th2 + Th3)*sin(Th5) - 0.5*(0.000115*cos(Th4)*sin(Th6) - 0.02603*sin(Th4)*sin(Th5) + 0.000115*cos(Th5)*cos(Th6)*sin(Th4))*(0.126*cos(Th2 + Th3) + 0.05206*cos(Th2 + Th3)*cos(Th5) + 0.254*cos(Th2)*cos(Th3) - 0.254*sin(Th2)*sin(Th3) + 0.00023*cos(Th2 + Th3)*cos(Th6)*sin(Th5) - 0.05206*sin(Th2 + Th3)*cos(Th4)*sin(Th5) - 0.00023*sin(Th2 + Th3)*sin(Th4)*sin(Th6) + 0.00023*sin(Th2 + Th3)*cos(Th4)*cos(Th5)*cos(Th6)) - 0.00002*cos(Th2 + Th3)*cos(Th4)*cos(Th5) + 2.0e-6*cos(Th2 + Th3)*cos(Th6)*sin(Th4) - 0.0051115*sin(Th2 + Th3)*cos(Th4)*sin(Th4) - 2.0e-6*sin(Th2 + Th3)*sin(Th5)*sin(Th6) + 0.00004*sin(Th2 + Th3)*cos(Th4)^2*sin(Th5) - 2.0e-6*cos(Th2 + Th3)*cos(Th4)*cos(Th5)*sin(Th6) + 0.0026665*cos(Th2 + Th3)*cos(Th5)*sin(Th4)*sin(Th5) - 1.5e-6*sin(Th2 + Th3)*cos(Th5)*cos(Th6)*sin(Th6) - 4.0e-6*cos(Th2 + Th3)*cos(Th5)^2*cos(Th6)*sin(Th4) + 0.0026665*sin(Th2 + Th3)*cos(Th4)*cos(Th5)^2*sin(Th4) + 1.5e-6*sin(Th2 + Th3)*cos(Th4)*cos(Th6)^2*sin(Th4) + 4.0e-6*sin(Th2 + Th3)*cos(Th4)^2*sin(Th5)*sin(Th6) + 1.5e-6*cos(Th2 + Th3)*cos(Th5)*cos(Th6)^2*sin(Th4)*sin(Th5) + 3.0e-6*sin(Th2 + Th3)*cos(Th4)^2*cos(Th5)*cos(Th6)*sin(Th6) + 1.5e-6*sin(Th2 + Th3)*cos(Th4)*cos(Th5)^2*cos(Th6)^2*sin(Th4) + 1.5e-6*cos(Th2 + Th3)*cos(Th4)*cos(Th6)*sin(Th5)*sin(Th6) + 4.0e-6*sin(Th2 + Th3)*cos(Th4)*cos(Th5)*cos(Th6)*sin(Th4)*sin(Th5))*dTh3*dTh1;
V332=(3.6e-6*cos(Th3)*sin(Th5) - 0.0028836*sin(Th3) - 0.0044118*cos(Th3)*cos(Th5) - 0.057271*cos(Th3) + 0.0001116*sin(Th3)*sin(Th4) + 3.6e-6*cos(Th4)*cos(Th5)*sin(Th3) - 0.0000207*cos(Th3)*cos(Th6)*sin(Th5) + 0.0044118*cos(Th4)*sin(Th3)*sin(Th5) + 0.0000207*sin(Th3)*sin(Th4)*sin(Th6) - 0.0000207*cos(Th4)*cos(Th5)*cos(Th6)*sin(Th3))*dTh3*dTh2;
V333=(0)*dTh3*dTh3;
V334=(4.96e-8*cos(Th4)^2*cos(Th5) - 2.48e-8*cos(Th5) - 0.000078115*sin(Th5) - 0.01158*sin(2.0*Th4) + 0.00015623*cos(Th4)^2*sin(Th5) - 0.000019974*sin(Th5)*sin(Th6) + 0.000039948*cos(Th4)^2*sin(Th5)*sin(Th6) - 5.9471e-6*cos(Th5)*cos(Th6)*sin(Th6) + 0.013381*cos(Th4)*cos(Th5)^2*sin(Th4) + 5.9471e-6*cos(Th4)*cos(Th6)^2*sin(Th4) + 5.9471e-6*cos(Th4)*cos(Th5)^2*cos(Th6)^2*sin(Th4) + 1.216e-7*cos(Th4)*cos(Th5)*sin(Th4)*sin(Th5) + 0.000011894*cos(Th4)^2*cos(Th5)*cos(Th6)*sin(Th6) + 0.000039948*cos(Th4)*cos(Th5)*cos(Th6)*sin(Th4)*sin(Th5))*dTh3*dTh4;
V335=(6.08e-8*cos(Th4)^2 - 0.0000152*cos(Th5) - 0.000019974*cos(Th6) - 0.018628*sin(Th5) - 0.0066904*sin(2.0*Th5) + 1.216e-7*cos(Th5)^2 + 0.000019974*cos(Th4)^2*cos(Th6) + 0.000039948*cos(Th5)^2*cos(Th6) - 1.216e-7*cos(Th4)^2*cos(Th5)^2 + 0.0000874*cos(Th5)*cos(Th6) - 0.000039948*cos(Th4)^2*cos(Th5)^2*cos(Th6) + 0.000078115*cos(Th4)*cos(Th5)*sin(Th4) - 2.48e-8*cos(Th4)*sin(Th4)*sin(Th5) + 0.013381*cos(Th4)^2*cos(Th5)*sin(Th5) - 5.9471e-6*cos(Th5)*cos(Th6)^2*sin(Th5) + 5.9471e-6*cos(Th4)^2*cos(Th5)*cos(Th6)^2*sin(Th5) + 0.000019974*cos(Th4)*cos(Th5)*sin(Th4)*sin(Th6) - 5.9471e-6*cos(Th4)*cos(Th6)*sin(Th4)*sin(Th5)*sin(Th6) - 6.08e-8)*dTh3*dTh5;
V336=(5.9471e-6*cos(Th4)^2*cos(Th6)*sin(Th6) - 5.9471e-6*cos(Th4)*cos(Th5)*sin(Th4) - 0.000019974*cos(Th5)*sin(Th5)*sin(Th6) - 0.0000874*sin(Th5)*sin(Th6) - 5.9471e-6*cos(Th5)^2*cos(Th6)*sin(Th6) + 5.9471e-6*cos(Th4)^2*cos(Th5)^2*cos(Th6)*sin(Th6) + 0.000019974*cos(Th4)*cos(Th6)*sin(Th4)*sin(Th5) + 0.000011894*cos(Th4)*cos(Th5)*cos(Th6)^2*sin(Th4) + 0.000019974*cos(Th4)^2*cos(Th5)*sin(Th5)*sin(Th6))*dTh3*dTh6;
%---------------------------
V341=(0.0061194*sin(Th2)*sin(Th3) - 0.0061194*cos(Th2)*cos(Th3) - 0.0033452*cos(Th5)^2*sin(Th2)*sin(Th3) + 1.4868e-6*cos(Th6)^2*sin(Th2)*sin(Th3) - 1.52e-8*cos(Th2)*cos(Th4)*sin(Th3) - 1.52e-8*cos(Th3)*cos(Th4)*sin(Th2) - 0.0001178*cos(Th2)*sin(Th3)*sin(Th4) - 0.0001178*cos(Th3)*sin(Th2)*sin(Th4) + 0.0033452*cos(Th2)*cos(Th3)*cos(Th5)^2 - 1.4868e-6*cos(Th2)*cos(Th3)*cos(Th6)^2 - 1.4868e-6*cos(Th5)^2*cos(Th6)^2*sin(Th2)*sin(Th3) - 3.8e-6*cos(Th2)*cos(Th4)*cos(Th5)*sin(Th3) - 3.8e-6*cos(Th3)*cos(Th4)*cos(Th5)*sin(Th2) + 3.04e-8*cos(Th2)*cos(Th3)*cos(Th5)*sin(Th5) - 4.9934e-6*cos(Th2)*cos(Th4)*cos(Th6)*sin(Th3) - 4.9934e-6*cos(Th3)*cos(Th4)*cos(Th6)*sin(Th2) - 0.0046569*cos(Th2)*cos(Th4)*sin(Th3)*sin(Th5) - 0.000019529*cos(Th2)*cos(Th5)*sin(Th3)*sin(Th4) - 0.0046569*cos(Th3)*cos(Th4)*sin(Th2)*sin(Th5) - 0.000019529*cos(Th3)*cos(Th5)*sin(Th2)*sin(Th4) + 6.2e-9*cos(Th2)*sin(Th3)*sin(Th4)*sin(Th5) + 6.2e-9*cos(Th3)*sin(Th2)*sin(Th4)*sin(Th5) - 0.00002185*cos(Th2)*sin(Th3)*sin(Th4)*sin(Th6) - 0.00002185*cos(Th3)*sin(Th2)*sin(Th4)*sin(Th6) - 3.04e-8*cos(Th5)*sin(Th2)*sin(Th3)*sin(Th5) + 3.04e-8*cos(Th2)*cos(Th4)*cos(Th5)^2*sin(Th3) + 3.04e-8*cos(Th3)*cos(Th4)*cos(Th5)^2*sin(Th2) + 1.4868e-6*cos(Th2)*cos(Th3)*cos(Th5)^2*cos(Th6)^2 + 0.00002185*cos(Th2)*cos(Th4)*cos(Th5)*cos(Th6)*sin(Th3) + 0.00002185*cos(Th3)*cos(Th4)*cos(Th5)*cos(Th6)*sin(Th2) + 9.9869e-6*cos(Th2)*cos(Th3)*cos(Th5)*cos(Th6)*sin(Th5) - 0.0033452*cos(Th2)*cos(Th4)*cos(Th5)*sin(Th3)*sin(Th5) - 0.0033452*cos(Th3)*cos(Th4)*cos(Th5)*sin(Th2)*sin(Th5) - 4.9934e-6*cos(Th2)*cos(Th5)*sin(Th3)*sin(Th4)*sin(Th6) - 4.9934e-6*cos(Th3)*cos(Th5)*sin(Th2)*sin(Th4)*sin(Th6) - 9.9869e-6*cos(Th5)*cos(Th6)*sin(Th2)*sin(Th3)*sin(Th5) + 9.9869e-6*cos(Th2)*cos(Th4)*cos(Th5)^2*cos(Th6)*sin(Th3) + 9.9869e-6*cos(Th3)*cos(Th4)*cos(Th5)^2*cos(Th6)*sin(Th2) - 1.4868e-6*cos(Th2)*cos(Th4)*cos(Th5)*cos(Th6)^2*sin(Th3)*sin(Th5) - 1.4868e-6*cos(Th3)*cos(Th4)*cos(Th5)*cos(Th6)^2*sin(Th2)*sin(Th5) + 1.4868e-6*cos(Th2)*cos(Th6)*sin(Th3)*sin(Th4)*sin(Th5)*sin(Th6) + 1.4868e-6*cos(Th3)*cos(Th6)*sin(Th2)*sin(Th4)*sin(Th5)*sin(Th6))*dTh4*dTh1;
V342=(-9.0e-7*cos(Th3)*(124.0*cos(Th4) - 4.0*cos(Th5)*sin(Th4) + 23.0*cos(Th4)*sin(Th6) - 4902.0*sin(Th4)*sin(Th5) + 23.0*cos(Th5)*cos(Th6)*sin(Th4)))*dTh4*dTh2;
V343=(0)*dTh4*dTh3;
V344=(6.08e-8*cos(Th4)*cos(Th5)^2 - 0.0002356*sin(Th4) - 3.04e-8*cos(Th4) - 7.6e-6*cos(Th4)*cos(Th5) - 9.9869e-6*cos(Th4)*cos(Th6) - 0.0093138*cos(Th4)*sin(Th5) - 0.000039058*cos(Th5)*sin(Th4) + 1.24e-8*sin(Th4)*sin(Th5) - 0.0000437*sin(Th4)*sin(Th6) + 4.0e-10*cos(Th2 + Th3)*sin(Th2 + Th3)*(31.0*cos(Th4) - 1.0*cos(Th5)*sin(Th4) + 76.0*sin(Th4)*sin(Th5))^2 + 0.0000437*cos(Th4)*cos(Th5)*cos(Th6) - 0.0066904*cos(Th4)*cos(Th5)*sin(Th5) - 9.9869e-6*cos(Th5)*sin(Th4)*sin(Th6) + 5.0e-11*cos(Th2 + Th3)*sin(Th2 + Th3)*(23.0*cos(Th4)*sin(Th6) - 5206.0*sin(Th4)*sin(Th5) + 23.0*cos(Th5)*cos(Th6)*sin(Th4))^2 + 0.000019974*cos(Th4)*cos(Th5)^2*cos(Th6) + cos(Th2 + Th3)*cos(Th1)*(0.00062*cos(Th4) - 0.00002*cos(Th5)*sin(Th4) + 0.00152*sin(Th4)*sin(Th5))*(0.00062*sin(Th1)*sin(Th4) - 0.00062*sin(Th2 + Th3)*cos(Th1)*cos(Th4) + 0.00002*cos(Th4)*cos(Th5)*sin(Th1) - 0.00152*cos(Th4)*sin(Th1)*sin(Th5) + 0.00002*sin(Th2 + Th3)*cos(Th1)*cos(Th5)*sin(Th4) - 0.00152*sin(Th2 + Th3)*cos(Th1)*sin(Th4)*sin(Th5)) + 2.9736e-6*cos(Th6)*sin(Th4)*sin(Th5)*sin(Th6) - 2.9736e-6*cos(Th4)*cos(Th5)*cos(Th6)^2*sin(Th5) + 0.5*cos(Th2 + Th3)*cos(Th1)*(0.00023*cos(Th4)*sin(Th6) - 0.05206*sin(Th4)*sin(Th5) + 0.00023*cos(Th5)*cos(Th6)*sin(Th4))*(0.05206*cos(Th4)*sin(Th1)*sin(Th5) + 0.00023*sin(Th1)*sin(Th4)*sin(Th6) - 0.00023*sin(Th2 + Th3)*cos(Th1)*cos(Th4)*sin(Th6) + 0.05206*sin(Th2 + Th3)*cos(Th1)*sin(Th4)*sin(Th5) - 0.00023*cos(Th4)*cos(Th5)*cos(Th6)*sin(Th1) - 0.00023*sin(Th2 + Th3)*cos(Th1)*cos(Th5)*cos(Th6)*sin(Th4)) - 0.5*cos(Th2 + Th3)*sin(Th1)*(0.00023*cos(Th4)*sin(Th6) - 0.05206*sin(Th4)*sin(Th5) + 0.00023*cos(Th5)*cos(Th6)*sin(Th4))*(0.05206*cos(Th1)*cos(Th4)*sin(Th5) + 0.00023*cos(Th1)*sin(Th4)*sin(Th6) + 0.00023*sin(Th2 + Th3)*cos(Th4)*sin(Th1)*sin(Th6) - 0.05206*sin(Th2 + Th3)*sin(Th1)*sin(Th4)*sin(Th5) - 0.00023*cos(Th1)*cos(Th4)*cos(Th5)*cos(Th6) + 0.00023*sin(Th2 + Th3)*cos(Th5)*cos(Th6)*sin(Th1)*sin(Th4)) - 1.0*cos(Th2 + Th3)*sin(Th1)*(0.00062*cos(Th4) - 0.00002*cos(Th5)*sin(Th4) + 0.00152*sin(Th4)*sin(Th5))*(0.00062*cos(Th1)*sin(Th4) + 0.00062*sin(Th2 + Th3)*cos(Th4)*sin(Th1) + 0.00002*cos(Th1)*cos(Th4)*cos(Th5) - 0.00152*cos(Th1)*cos(Th4)*sin(Th5) - 0.00002*sin(Th2 + Th3)*cos(Th5)*sin(Th1)*sin(Th4) + 0.00152*sin(Th2 + Th3)*sin(Th1)*sin(Th4)*sin(Th5)))*dTh4*dTh4;
V345=(7.6e-6*sin(Th4)*sin(Th5) - 0.000039058*cos(Th4)*sin(Th5) - 0.0093138*cos(Th5)*sin(Th4) - 1.24e-8*cos(Th4)*cos(Th5) - 0.0066919*sin(Th4)*(2.0*cos(Th5)^2 - 1.0) - 1.216e-7*cos(Th5)*sin(Th4)*sin(Th5) - 9.9869e-6*cos(Th4)*sin(Th5)*sin(Th6) - 0.0000437*cos(Th6)*sin(Th4)*sin(Th5) - 1.4868e-6*sin(Th4)*(2.0*cos(Th5)^2 - 1.0)*(2.0*cos(Th6)^2 - 1.0) - 2.9736e-6*cos(Th4)*cos(Th5)*cos(Th6)*sin(Th6) - 0.000039948*cos(Th5)*cos(Th6)*sin(Th4)*sin(Th5))*dTh4*dTh5;
V346=(0.0000437*cos(Th4)*cos(Th6) + 9.9869e-6*cos(Th4)*cos(Th5)*cos(Th6) - 0.0000437*cos(Th5)*sin(Th4)*sin(Th6) - 2.9736e-6*cos(Th4)*sin(Th5)*(2.0*cos(Th6)^2 - 1.0) - 9.9869e-6*sin(Th4)*sin(Th6)*(2.0*cos(Th5)^2 - 1.0) + 5.9471e-6*cos(Th5)*cos(Th6)*sin(Th4)*sin(Th5)*sin(Th6))*dTh4*dTh6;
%---------------------------
V351=(6.2e-9*cos(Th2)*cos(Th3)*sin(Th5) - 0.000019529*cos(Th2)*cos(Th3)*cos(Th5) - 0.0037962*cos(Th2)*sin(Th3)*sin(Th4) - 0.0037962*cos(Th3)*sin(Th2)*sin(Th4) + 0.000019529*cos(Th5)*sin(Th2)*sin(Th3) - 6.2e-9*sin(Th2)*sin(Th3)*sin(Th5) + 6.2e-9*cos(Th2)*cos(Th4)*cos(Th5)*sin(Th3) + 6.2e-9*cos(Th3)*cos(Th4)*cos(Th5)*sin(Th2) - 4.9934e-6*cos(Th2)*cos(Th3)*cos(Th5)*sin(Th6) + 0.000019529*cos(Th2)*cos(Th4)*sin(Th3)*sin(Th5) - 0.0046569*cos(Th2)*cos(Th5)*sin(Th3)*sin(Th4) + 0.000019529*cos(Th3)*cos(Th4)*sin(Th2)*sin(Th5) - 0.0046569*cos(Th3)*cos(Th5)*sin(Th2)*sin(Th4) + 3.8e-6*cos(Th2)*sin(Th3)*sin(Th4)*sin(Th5) + 3.8e-6*cos(Th3)*sin(Th2)*sin(Th4)*sin(Th5) + 4.9934e-6*cos(Th5)*sin(Th2)*sin(Th3)*sin(Th6) + 1.4868e-6*cos(Th2)*cos(Th6)^2*sin(Th3)*sin(Th4) + 1.4868e-6*cos(Th3)*cos(Th6)^2*sin(Th2)*sin(Th4) + 1.4868e-6*cos(Th2)*cos(Th3)*cos(Th6)*sin(Th5)*sin(Th6) + 4.9934e-6*cos(Th2)*cos(Th4)*sin(Th3)*sin(Th5)*sin(Th6) - 0.00002185*cos(Th2)*cos(Th6)*sin(Th3)*sin(Th4)*sin(Th5) + 4.9934e-6*cos(Th3)*cos(Th4)*sin(Th2)*sin(Th5)*sin(Th6) - 0.00002185*cos(Th3)*cos(Th6)*sin(Th2)*sin(Th4)*sin(Th5) - 1.4868e-6*cos(Th6)*sin(Th2)*sin(Th3)*sin(Th5)*sin(Th6) + 1.4868e-6*cos(Th2)*cos(Th4)*cos(Th5)*cos(Th6)*sin(Th3)*sin(Th6) + 1.4868e-6*cos(Th3)*cos(Th4)*cos(Th5)*cos(Th6)*sin(Th2)*sin(Th6))*dTh5*dTh1;
V352=(3.6e-6*cos(Th5)*sin(Th3) + 0.0044118*sin(Th3)*sin(Th5) - 0.0044118*cos(Th3)*cos(Th4)*cos(Th5) + 3.6e-6*cos(Th3)*cos(Th4)*sin(Th5) - 0.0000207*cos(Th5)*cos(Th6)*sin(Th3) - 0.0000207*cos(Th3)*cos(Th4)*cos(Th6)*sin(Th5))*dTh5*dTh2;
V353=(0)*dTh5*dTh3;
V354=(2.9736e-6*cos(Th6)^2*sin(Th4) - 0.0075924*sin(Th4) + 1.24e-8*cos(Th4)*cos(Th5) + 0.000039058*cos(Th4)*sin(Th5) - 0.0093138*cos(Th5)*sin(Th4) + 7.6e-6*sin(Th4)*sin(Th5) - 0.5*sin(Th2 + Th3)*(0.00062*cos(Th4) - 0.00002*cos(Th5)*sin(Th4) + 0.00152*sin(Th4)*sin(Th5))*(0.00002*sin(Th2 + Th3)*cos(Th5) - 0.00152*sin(Th2 + Th3)*sin(Th5) + 0.00152*cos(Th2 + Th3)*cos(Th4)*cos(Th5) + 0.00002*cos(Th2 + Th3)*cos(Th4)*sin(Th5)) - 0.5*cos(Th2 + Th3)*(0.00062*cos(Th4) - 0.00002*cos(Th5)*sin(Th4) + 0.00152*sin(Th4)*sin(Th5))*(0.00152*cos(Th2 + Th3)*sin(Th5) - 0.00002*cos(Th2 + Th3)*cos(Th5) + 0.00152*sin(Th2 + Th3)*cos(Th4)*cos(Th5) + 0.00002*sin(Th2 + Th3)*cos(Th4)*sin(Th5)) + 0.25*cos(Th2 + Th3)*(0.00023*cos(Th4)*sin(Th6) - 0.05206*sin(Th4)*sin(Th5) + 0.00023*cos(Th5)*cos(Th6)*sin(Th4))*(0.05206*cos(Th2 + Th3)*sin(Th5) - 0.00023*cos(Th2 + Th3)*cos(Th5)*cos(Th6) + 0.05206*sin(Th2 + Th3)*cos(Th4)*cos(Th5) + 0.00023*sin(Th2 + Th3)*cos(Th4)*cos(Th6)*sin(Th5)) + 0.25*cos(Th1)*(0.05206*cos(Th2 + Th3)*cos(Th4)*cos(Th5) - 0.05206*sin(Th2 + Th3)*sin(Th5) + 0.00023*sin(Th2 + Th3)*cos(Th5)*cos(Th6) + 0.00023*cos(Th2 + Th3)*cos(Th4)*cos(Th6)*sin(Th5))*(0.05206*cos(Th4)*sin(Th1)*sin(Th5) + 0.00023*sin(Th1)*sin(Th4)*sin(Th6) - 0.00023*sin(Th2 + Th3)*cos(Th1)*cos(Th4)*sin(Th6) + 0.05206*sin(Th2 + Th3)*cos(Th1)*sin(Th4)*sin(Th5) - 0.00023*cos(Th4)*cos(Th5)*cos(Th6)*sin(Th1) - 0.00023*sin(Th2 + Th3)*cos(Th1)*cos(Th5)*cos(Th6)*sin(Th4)) + 0.5*sin(Th1)*(0.00002*sin(Th2 + Th3)*cos(Th5) - 0.00152*sin(Th2 + Th3)*sin(Th5) + 0.00152*cos(Th2 + Th3)*cos(Th4)*cos(Th5) + 0.00002*cos(Th2 + Th3)*cos(Th4)*sin(Th5))*(0.00062*cos(Th1)*sin(Th4) + 0.00062*sin(Th2 + Th3)*cos(Th4)*sin(Th1) + 0.00002*cos(Th1)*cos(Th4)*cos(Th5) - 0.00152*cos(Th1)*cos(Th4)*sin(Th5) - 0.00002*sin(Th2 + Th3)*cos(Th5)*sin(Th1)*sin(Th4) + 0.00152*sin(Th2 + Th3)*sin(Th1)*sin(Th4)*sin(Th5)) - 0.25*sin(Th1)*(0.05206*cos(Th2 + Th3)*cos(Th4)*cos(Th5) - 0.05206*sin(Th2 + Th3)*sin(Th5) + 0.00023*sin(Th2 + Th3)*cos(Th5)*cos(Th6) + 0.00023*cos(Th2 + Th3)*cos(Th4)*cos(Th6)*sin(Th5))*(0.05206*cos(Th1)*cos(Th4)*sin(Th5) + 0.00023*cos(Th1)*sin(Th4)*sin(Th6) + 0.00023*sin(Th2 + Th3)*cos(Th4)*sin(Th1)*sin(Th6) - 0.05206*sin(Th2 + Th3)*sin(Th1)*sin(Th4)*sin(Th5) - 0.00023*cos(Th1)*cos(Th4)*cos(Th5)*cos(Th6) + 0.00023*sin(Th2 + Th3)*cos(Th5)*cos(Th6)*sin(Th1)*sin(Th4)) + 0.25*sin(Th2 + Th3)*(0.00023*cos(Th4)*sin(Th6) - 0.05206*sin(Th4)*sin(Th5) + 0.00023*cos(Th5)*cos(Th6)*sin(Th4))*(0.05206*cos(Th2 + Th3)*cos(Th4)*cos(Th5) - 0.05206*sin(Th2 + Th3)*sin(Th5) + 0.00023*sin(Th2 + Th3)*cos(Th5)*cos(Th6) + 0.00023*cos(Th2 + Th3)*cos(Th4)*cos(Th6)*sin(Th5)) + 9.9869e-6*cos(Th4)*sin(Th5)*sin(Th6) - 0.0000437*cos(Th6)*sin(Th4)*sin(Th5) - 0.5*cos(Th1)*(0.00002*sin(Th2 + Th3)*cos(Th5) - 0.00152*sin(Th2 + Th3)*sin(Th5) + 0.00152*cos(Th2 + Th3)*cos(Th4)*cos(Th5) + 0.00002*cos(Th2 + Th3)*cos(Th4)*sin(Th5))*(0.00062*sin(Th1)*sin(Th4) - 0.00062*sin(Th2 + Th3)*cos(Th1)*cos(Th4) + 0.00002*cos(Th4)*cos(Th5)*sin(Th1) - 0.00152*cos(Th4)*sin(Th1)*sin(Th5) + 0.00002*sin(Th2 + Th3)*cos(Th1)*cos(Th5)*sin(Th4) - 0.00152*sin(Th2 + Th3)*cos(Th1)*sin(Th4)*sin(Th5)) + 0.5*cos(Th2 + Th3)*sin(Th1)*(0.00062*cos(Th4) - 0.00002*cos(Th5)*sin(Th4) + 0.00152*sin(Th4)*sin(Th5))*(0.00152*cos(Th2 + Th3)*sin(Th1)*sin(Th5) - 0.00002*cos(Th2 + Th3)*cos(Th5)*sin(Th1) + 0.00152*cos(Th1)*cos(Th5)*sin(Th4) + 0.00002*cos(Th1)*sin(Th4)*sin(Th5) + 0.00152*sin(Th2 + Th3)*cos(Th4)*cos(Th5)*sin(Th1) + 0.00002*sin(Th2 + Th3)*cos(Th4)*sin(Th1)*sin(Th5)) - 0.25*cos(Th2 + Th3)*sin(Th1)*(0.00023*cos(Th4)*sin(Th6) - 0.05206*sin(Th4)*sin(Th5) + 0.00023*cos(Th5)*cos(Th6)*sin(Th4))*(0.05206*cos(Th2 + Th3)*sin(Th1)*sin(Th5) + 0.05206*cos(Th1)*cos(Th5)*sin(Th4) - 0.00023*cos(Th2 + Th3)*cos(Th5)*cos(Th6)*sin(Th1) + 0.05206*sin(Th2 + Th3)*cos(Th4)*cos(Th5)*sin(Th1) + 0.00023*cos(Th1)*cos(Th6)*sin(Th4)*sin(Th5) + 0.00023*sin(Th2 + Th3)*cos(Th4)*cos(Th6)*sin(Th1)*sin(Th5)) - 0.25*cos(Th2 + Th3)*cos(Th1)*(0.00023*cos(Th4)*sin(Th6) - 0.05206*sin(Th4)*sin(Th5) + 0.00023*cos(Th5)*cos(Th6)*sin(Th4))*(0.05206*cos(Th2 + Th3)*cos(Th1)*sin(Th5) - 0.05206*cos(Th5)*sin(Th1)*sin(Th4) + 0.05206*sin(Th2 + Th3)*cos(Th1)*cos(Th4)*cos(Th5) - 0.00023*cos(Th6)*sin(Th1)*sin(Th4)*sin(Th5) - 0.00023*cos(Th2 + Th3)*cos(Th1)*cos(Th5)*cos(Th6) + 0.00023*sin(Th2 + Th3)*cos(Th1)*cos(Th4)*cos(Th6)*sin(Th5)) + 2.9736e-6*cos(Th4)*cos(Th5)*cos(Th6)*sin(Th6) - 0.5*cos(Th2 + Th3)*cos(Th1)*(0.00062*cos(Th4) - 0.00002*cos(Th5)*sin(Th4) + 0.00152*sin(Th4)*sin(Th5))*(0.00002*cos(Th2 + Th3)*cos(Th1)*cos(Th5) - 0.00152*cos(Th2 + Th3)*cos(Th1)*sin(Th5) + 0.00152*cos(Th5)*sin(Th1)*sin(Th4) + 0.00002*sin(Th1)*sin(Th4)*sin(Th5) - 0.00152*sin(Th2 + Th3)*cos(Th1)*cos(Th4)*cos(Th5) - 0.00002*sin(Th2 + Th3)*cos(Th1)*cos(Th4)*sin(Th5)))*dTh5*dTh4;
V355=((0.00002*sin(Th2 + Th3)*cos(Th5) - 0.00152*sin(Th2 + Th3)*sin(Th5) + 0.00152*cos(Th2 + Th3)*cos(Th4)*cos(Th5) + 0.00002*cos(Th2 + Th3)*cos(Th4)*sin(Th5))*(0.00152*cos(Th2 + Th3)*sin(Th5) - 0.00002*cos(Th2 + Th3)*cos(Th5) + 0.00152*sin(Th2 + Th3)*cos(Th4)*cos(Th5) + 0.00002*sin(Th2 + Th3)*cos(Th4)*sin(Th5)) + (0.02603*cos(Th2 + Th3)*sin(Th5) - 0.000115*cos(Th2 + Th3)*cos(Th5)*cos(Th6) + 0.02603*sin(Th2 + Th3)*cos(Th4)*cos(Th5) + 0.000115*sin(Th2 + Th3)*cos(Th4)*cos(Th6)*sin(Th5))*(0.05206*cos(Th2 + Th3)*cos(Th4)*cos(Th5) - 0.05206*sin(Th2 + Th3)*sin(Th5) + 0.00023*sin(Th2 + Th3)*cos(Th5)*cos(Th6) + 0.00023*cos(Th2 + Th3)*cos(Th4)*cos(Th6)*sin(Th5)) - 7.6e-6*cos(Th4)*cos(Th5) - 0.0093138*cos(Th4)*sin(Th5) + 0.000039058*cos(Th5)*sin(Th4) - 1.24e-8*sin(Th4)*sin(Th5) - 0.5*cos(Th1)*(0.05206*cos(Th2 + Th3)*cos(Th4)*cos(Th5) - 0.05206*sin(Th2 + Th3)*sin(Th5) + 0.00023*sin(Th2 + Th3)*cos(Th5)*cos(Th6) + 0.00023*cos(Th2 + Th3)*cos(Th4)*cos(Th6)*sin(Th5))*(0.05206*cos(Th2 + Th3)*cos(Th1)*sin(Th5) - 0.05206*cos(Th5)*sin(Th1)*sin(Th4) + 0.05206*sin(Th2 + Th3)*cos(Th1)*cos(Th4)*cos(Th5) - 0.00023*cos(Th6)*sin(Th1)*sin(Th4)*sin(Th5) - 0.00023*cos(Th2 + Th3)*cos(Th1)*cos(Th5)*cos(Th6) + 0.00023*sin(Th2 + Th3)*cos(Th1)*cos(Th4)*cos(Th6)*sin(Th5)) + cos(Th1)*(0.00002*sin(Th2 + Th3)*cos(Th5) - 0.00152*sin(Th2 + Th3)*sin(Th5) + 0.00152*cos(Th2 + Th3)*cos(Th4)*cos(Th5) + 0.00002*cos(Th2 + Th3)*cos(Th4)*sin(Th5))*(0.00002*cos(Th2 + Th3)*cos(Th1)*cos(Th5) - 0.00152*cos(Th2 + Th3)*cos(Th1)*sin(Th5) + 0.00152*cos(Th5)*sin(Th1)*sin(Th4) + 0.00002*sin(Th1)*sin(Th4)*sin(Th5) - 0.00152*sin(Th2 + Th3)*cos(Th1)*cos(Th4)*cos(Th5) - 0.00002*sin(Th2 + Th3)*cos(Th1)*cos(Th4)*sin(Th5)) + 2.7105e-25*sin(Th4)*sin(Th6)*(1.4757e19*cos(Th5) - 1.1068e19*cos(Th6)*sin(Th5)) + 0.0000437*cos(Th4)*cos(Th5)*cos(Th6) + 5.9869e-6*cos(Th5)*sin(Th4)*sin(Th6) - 1.0*sin(Th1)*(0.00002*sin(Th2 + Th3)*cos(Th5) - 0.00152*sin(Th2 + Th3)*sin(Th5) + 0.00152*cos(Th2 + Th3)*cos(Th4)*cos(Th5) + 0.00002*cos(Th2 + Th3)*cos(Th4)*sin(Th5))*(0.00152*cos(Th2 + Th3)*sin(Th1)*sin(Th5) - 0.00002*cos(Th2 + Th3)*cos(Th5)*sin(Th1) + 0.00152*cos(Th1)*cos(Th5)*sin(Th4) + 0.00002*cos(Th1)*sin(Th4)*sin(Th5) + 0.00152*sin(Th2 + Th3)*cos(Th4)*cos(Th5)*sin(Th1) + 0.00002*sin(Th2 + Th3)*cos(Th4)*sin(Th1)*sin(Th5)) - 0.5*sin(Th1)*(0.05206*cos(Th2 + Th3)*cos(Th4)*cos(Th5) - 0.05206*sin(Th2 + Th3)*sin(Th5) + 0.00023*sin(Th2 + Th3)*cos(Th5)*cos(Th6) + 0.00023*cos(Th2 + Th3)*cos(Th4)*cos(Th6)*sin(Th5))*(0.05206*cos(Th2 + Th3)*sin(Th1)*sin(Th5) + 0.05206*cos(Th1)*cos(Th5)*sin(Th4) - 0.00023*cos(Th2 + Th3)*cos(Th5)*cos(Th6)*sin(Th1) + 0.05206*sin(Th2 + Th3)*cos(Th4)*cos(Th5)*sin(Th1) + 0.00023*cos(Th1)*cos(Th6)*sin(Th4)*sin(Th5) + 0.00023*sin(Th2 + Th3)*cos(Th4)*cos(Th6)*sin(Th1)*sin(Th5)) + 2.645e-8*cos(Th6)*sin(Th4)*sin(Th5)*sin(Th6))*dTh5*dTh5;
V356=(5.9471e-6*cos(Th4)*cos(Th6)*sin(Th6) - 0.0000437*cos(Th4)*sin(Th5)*sin(Th6) + 9.9869e-6*cos(Th6)*sin(Th4)*sin(Th5) + 2.9736e-6*cos(Th5)*sin(Th4)*(2.0*cos(Th6)^2 - 1.0))*dTh5*dTh6;
%---------------------------
V361=(0.000058013*cos(Th5)*sin(Th2)*sin(Th3) - 0.000058013*cos(Th2)*cos(Th3)*cos(Th5) + 0.00002185*cos(Th2)*cos(Th4)*cos(Th6)*sin(Th3) + 0.00002185*cos(Th3)*cos(Th4)*cos(Th6)*sin(Th2) + 4.9934e-6*cos(Th2)*cos(Th3)*cos(Th6)*sin(Th5) + 0.000058013*cos(Th2)*cos(Th4)*sin(Th3)*sin(Th5) + 0.000058013*cos(Th3)*cos(Th4)*sin(Th2)*sin(Th5) - 4.9934e-6*cos(Th2)*sin(Th3)*sin(Th4)*sin(Th6) - 4.9934e-6*cos(Th3)*sin(Th2)*sin(Th4)*sin(Th6) - 4.9934e-6*cos(Th6)*sin(Th2)*sin(Th3)*sin(Th5) + 4.9934e-6*cos(Th2)*cos(Th4)*cos(Th5)*cos(Th6)*sin(Th3) + 4.9934e-6*cos(Th3)*cos(Th4)*cos(Th5)*cos(Th6)*sin(Th2) - 0.00002185*cos(Th2)*cos(Th5)*sin(Th3)*sin(Th4)*sin(Th6) - 0.00002185*cos(Th3)*cos(Th5)*sin(Th2)*sin(Th4)*sin(Th6))*dTh6*dTh1;
V362=(0.0000207*sin(Th3)*sin(Th5)*sin(Th6) - 0.0000207*cos(Th3)*cos(Th6)*sin(Th4) - 0.0000207*cos(Th3)*cos(Th4)*cos(Th5)*sin(Th6))*dTh6*dTh2;
V363=(0)*dTh6*dTh3;
V364=(0.0000437*cos(Th4)*cos(Th6) + 0.00011603*cos(Th4)*sin(Th5) - 9.9869e-6*sin(Th4)*sin(Th6) + 9.9869e-6*cos(Th4)*cos(Th5)*cos(Th6) + 0.25*cos(Th1)*(0.00023*cos(Th2 + Th3)*cos(Th6)*sin(Th4) - 0.00023*sin(Th2 + Th3)*sin(Th5)*sin(Th6) + 0.00023*cos(Th2 + Th3)*cos(Th4)*cos(Th5)*sin(Th6))*(0.05206*cos(Th4)*sin(Th1)*sin(Th5) + 0.00023*sin(Th1)*sin(Th4)*sin(Th6) - 0.00023*sin(Th2 + Th3)*cos(Th1)*cos(Th4)*sin(Th6) + 0.05206*sin(Th2 + Th3)*cos(Th1)*sin(Th4)*sin(Th5) - 0.00023*cos(Th4)*cos(Th5)*cos(Th6)*sin(Th1) - 0.00023*sin(Th2 + Th3)*cos(Th1)*cos(Th5)*cos(Th6)*sin(Th4)) - 0.0000437*cos(Th5)*sin(Th4)*sin(Th6) + 0.25*cos(Th2 + Th3)*(0.00023*cos(Th4)*sin(Th6) - 0.05206*sin(Th4)*sin(Th5) + 0.00023*cos(Th5)*cos(Th6)*sin(Th4))*(0.00023*sin(Th2 + Th3)*cos(Th6)*sin(Th4) + 0.00023*cos(Th2 + Th3)*sin(Th5)*sin(Th6) + 0.00023*sin(Th2 + Th3)*cos(Th4)*cos(Th5)*sin(Th6)) - 0.25*sin(Th1)*(0.00023*cos(Th2 + Th3)*cos(Th6)*sin(Th4) - 0.00023*sin(Th2 + Th3)*sin(Th5)*sin(Th6) + 0.00023*cos(Th2 + Th3)*cos(Th4)*cos(Th5)*sin(Th6))*(0.05206*cos(Th1)*cos(Th4)*sin(Th5) + 0.00023*cos(Th1)*sin(Th4)*sin(Th6) + 0.00023*sin(Th2 + Th3)*cos(Th4)*sin(Th1)*sin(Th6) - 0.05206*sin(Th2 + Th3)*sin(Th1)*sin(Th4)*sin(Th5) - 0.00023*cos(Th1)*cos(Th4)*cos(Th5)*cos(Th6) + 0.00023*sin(Th2 + Th3)*cos(Th5)*cos(Th6)*sin(Th1)*sin(Th4)) + 0.25*sin(Th2 + Th3)*(0.00023*cos(Th4)*sin(Th6) - 0.05206*sin(Th4)*sin(Th5) + 0.00023*cos(Th5)*cos(Th6)*sin(Th4))*(0.00023*cos(Th2 + Th3)*cos(Th6)*sin(Th4) - 0.00023*sin(Th2 + Th3)*sin(Th5)*sin(Th6) + 0.00023*cos(Th2 + Th3)*cos(Th4)*cos(Th5)*sin(Th6)) - 0.25*cos(Th2 + Th3)*cos(Th1)*(0.00023*cos(Th4)*sin(Th6) - 0.05206*sin(Th4)*sin(Th5) + 0.00023*cos(Th5)*cos(Th6)*sin(Th4))*(0.00023*cos(Th4)*cos(Th6)*sin(Th1) + 0.00023*sin(Th2 + Th3)*cos(Th1)*cos(Th6)*sin(Th4) + 0.00023*cos(Th2 + Th3)*cos(Th1)*sin(Th5)*sin(Th6) - 0.00023*cos(Th5)*sin(Th1)*sin(Th4)*sin(Th6) + 0.00023*sin(Th2 + Th3)*cos(Th1)*cos(Th4)*cos(Th5)*sin(Th6)) - 0.25*cos(Th2 + Th3)*sin(Th1)*(0.00023*cos(Th4)*sin(Th6) - 0.05206*sin(Th4)*sin(Th5) + 0.00023*cos(Th5)*cos(Th6)*sin(Th4))*(0.00023*sin(Th2 + Th3)*cos(Th6)*sin(Th1)*sin(Th4) - 0.00023*cos(Th1)*cos(Th4)*cos(Th6) + 0.00023*cos(Th2 + Th3)*sin(Th1)*sin(Th5)*sin(Th6) + 0.00023*cos(Th1)*cos(Th5)*sin(Th4)*sin(Th6) + 0.00023*sin(Th2 + Th3)*cos(Th4)*cos(Th5)*sin(Th1)*sin(Th6)))*dTh6*dTh4;
V365=(0.5*(0.000115*cos(Th2 + Th3)*cos(Th6)*sin(Th4) - 0.000115*sin(Th2 + Th3)*sin(Th5)*sin(Th6) + 0.000115*cos(Th2 + Th3)*cos(Th4)*cos(Th5)*sin(Th6))*(0.05206*cos(Th2 + Th3)*sin(Th5) - 0.00023*cos(Th2 + Th3)*cos(Th5)*cos(Th6) + 0.05206*sin(Th2 + Th3)*cos(Th4)*cos(Th5) + 0.00023*sin(Th2 + Th3)*cos(Th4)*cos(Th6)*sin(Th5)) + 0.5*(0.000115*sin(Th2 + Th3)*cos(Th6)*sin(Th4) + 0.000115*cos(Th2 + Th3)*sin(Th5)*sin(Th6) + 0.000115*sin(Th2 + Th3)*cos(Th4)*cos(Th5)*sin(Th6))*(0.05206*cos(Th2 + Th3)*cos(Th4)*cos(Th5) - 0.05206*sin(Th2 + Th3)*sin(Th5) + 0.00023*sin(Th2 + Th3)*cos(Th5)*cos(Th6) + 0.00023*cos(Th2 + Th3)*cos(Th4)*cos(Th6)*sin(Th5)) + sin(Th4)*(0.000116*cos(Th5) - 4.0e-6*cos(Th6)*sin(Th5)) + 2.645e-8*cos(Th5)*sin(Th4) - 0.25*sin(Th1)*(0.00023*cos(Th2 + Th3)*cos(Th6)*sin(Th4) - 0.00023*sin(Th2 + Th3)*sin(Th5)*sin(Th6) + 0.00023*cos(Th2 + Th3)*cos(Th4)*cos(Th5)*sin(Th6))*(0.05206*cos(Th2 + Th3)*sin(Th1)*sin(Th5) + 0.05206*cos(Th1)*cos(Th5)*sin(Th4) - 0.00023*cos(Th2 + Th3)*cos(Th5)*cos(Th6)*sin(Th1) + 0.05206*sin(Th2 + Th3)*cos(Th4)*cos(Th5)*sin(Th1) + 0.00023*cos(Th1)*cos(Th6)*sin(Th4)*sin(Th5) + 0.00023*sin(Th2 + Th3)*cos(Th4)*cos(Th6)*sin(Th1)*sin(Th5)) - 0.25*cos(Th1)*(0.00023*cos(Th2 + Th3)*cos(Th6)*sin(Th4) - 0.00023*sin(Th2 + Th3)*sin(Th5)*sin(Th6) + 0.00023*cos(Th2 + Th3)*cos(Th4)*cos(Th5)*sin(Th6))*(0.05206*cos(Th2 + Th3)*cos(Th1)*sin(Th5) - 0.05206*cos(Th5)*sin(Th1)*sin(Th4) + 0.05206*sin(Th2 + Th3)*cos(Th1)*cos(Th4)*cos(Th5) - 0.00023*cos(Th6)*sin(Th1)*sin(Th4)*sin(Th5) - 0.00023*cos(Th2 + Th3)*cos(Th1)*cos(Th5)*cos(Th6) + 0.00023*sin(Th2 + Th3)*cos(Th1)*cos(Th4)*cos(Th6)*sin(Th5)) - 0.25*cos(Th1)*(0.05206*cos(Th2 + Th3)*cos(Th4)*cos(Th5) - 0.05206*sin(Th2 + Th3)*sin(Th5) + 0.00023*sin(Th2 + Th3)*cos(Th5)*cos(Th6) + 0.00023*cos(Th2 + Th3)*cos(Th4)*cos(Th6)*sin(Th5))*(0.00023*cos(Th4)*cos(Th6)*sin(Th1) + 0.00023*sin(Th2 + Th3)*cos(Th1)*cos(Th6)*sin(Th4) + 0.00023*cos(Th2 + Th3)*cos(Th1)*sin(Th5)*sin(Th6) - 0.00023*cos(Th5)*sin(Th1)*sin(Th4)*sin(Th6) + 0.00023*sin(Th2 + Th3)*cos(Th1)*cos(Th4)*cos(Th5)*sin(Th6)) - 0.25*sin(Th1)*(0.05206*cos(Th2 + Th3)*cos(Th4)*cos(Th5) - 0.05206*sin(Th2 + Th3)*sin(Th5) + 0.00023*sin(Th2 + Th3)*cos(Th5)*cos(Th6) + 0.00023*cos(Th2 + Th3)*cos(Th4)*cos(Th6)*sin(Th5))*(0.00023*sin(Th2 + Th3)*cos(Th6)*sin(Th1)*sin(Th4) - 0.00023*cos(Th1)*cos(Th4)*cos(Th6) + 0.00023*cos(Th2 + Th3)*sin(Th1)*sin(Th5)*sin(Th6) + 0.00023*cos(Th1)*cos(Th5)*sin(Th4)*sin(Th6) + 0.00023*sin(Th2 + Th3)*cos(Th4)*cos(Th5)*sin(Th1)*sin(Th6)) - 0.0000437*cos(Th4)*sin(Th5)*sin(Th6) - 5.9869e-6*cos(Th6)*sin(Th4)*sin(Th5))*dTh6*dTh5;
V366=((0.000115*cos(Th2 + Th3)*cos(Th6)*sin(Th4) - 0.000115*sin(Th2 + Th3)*sin(Th5)*sin(Th6) + 0.000115*cos(Th2 + Th3)*cos(Th4)*cos(Th5)*sin(Th6))*(0.00023*sin(Th2 + Th3)*cos(Th6)*sin(Th4) + 0.00023*cos(Th2 + Th3)*sin(Th5)*sin(Th6) + 0.00023*sin(Th2 + Th3)*cos(Th4)*cos(Th5)*sin(Th6)) + 9.9869e-6*cos(Th4)*cos(Th6) - 0.0000437*sin(Th4)*sin(Th6) - 0.5*cos(Th1)*(0.00023*cos(Th2 + Th3)*cos(Th6)*sin(Th4) - 0.00023*sin(Th2 + Th3)*sin(Th5)*sin(Th6) + 0.00023*cos(Th2 + Th3)*cos(Th4)*cos(Th5)*sin(Th6))*(0.00023*cos(Th4)*cos(Th6)*sin(Th1) + 0.00023*sin(Th2 + Th3)*cos(Th1)*cos(Th6)*sin(Th4) + 0.00023*cos(Th2 + Th3)*cos(Th1)*sin(Th5)*sin(Th6) - 0.00023*cos(Th5)*sin(Th1)*sin(Th4)*sin(Th6) + 0.00023*sin(Th2 + Th3)*cos(Th1)*cos(Th4)*cos(Th5)*sin(Th6)) - 0.5*sin(Th1)*(0.00023*cos(Th2 + Th3)*cos(Th6)*sin(Th4) - 0.00023*sin(Th2 + Th3)*sin(Th5)*sin(Th6) + 0.00023*cos(Th2 + Th3)*cos(Th4)*cos(Th5)*sin(Th6))*(0.00023*sin(Th2 + Th3)*cos(Th6)*sin(Th1)*sin(Th4) - 0.00023*cos(Th1)*cos(Th4)*cos(Th6) + 0.00023*cos(Th2 + Th3)*sin(Th1)*sin(Th5)*sin(Th6) + 0.00023*cos(Th1)*cos(Th5)*sin(Th4)*sin(Th6) + 0.00023*sin(Th2 + Th3)*cos(Th4)*cos(Th5)*sin(Th1)*sin(Th6)) + 0.0000437*cos(Th4)*cos(Th5)*cos(Th6) - 9.9869e-6*cos(Th5)*sin(Th4)*sin(Th6))*dTh6*dTh6;
%---------------------------
V3 = V311+V312+V313+V314+V315+V316+V321+V322+V323+V324+V325+V326+...
     V331+V332+V333+V334+V335+V336+V341+V342+V343+V344+V345+V346+...
     V351+V352+V353+V354+V355+V356+V361+V362+V363+V364+V365+V366;
end
